simulink model "CanonicalMax"  (R2020a)
settings: Solver=VariableStepAuto  StartTime=0.0  StopTime=20  RelTol=1e-3
settings Model: Creator=Lenovo  LastModifiedBy=Lenovo

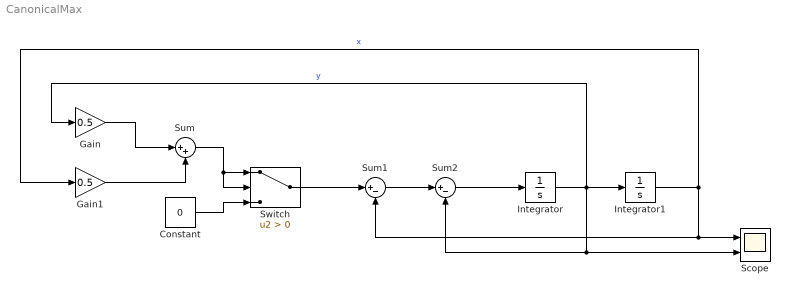
== system CanonicalMax ==
  Constant : Constant  Value=0
  Gain : Gain  Gain=0.5
  Gain1 : Gain  Gain=0.5
  Integrator : Integrator  InitialCondition=1
  Integrator1 : Integrator  InitialCondition=1
  Scope : Scope  NumInputPorts=2
  Sum : Sum  Inputs=|++
  Sum1 : Sum  Inputs=|+-
  Sum2 : Sum  Inputs=|+-
  Switch : Switch  Criteria=u2 > Threshold
  wires:
  Gain/1 -> Sum/1
  Gain1/1 -> Sum/2
  Sum1/1 -> Sum2/1
  Sum2/1 -> Integrator/1
  Integrator/1 -> Gain/1, Scope/2, Sum2/2, Integrator1/1  "y"
  Integrator1/1 -> Sum1/2, Scope/1, Gain1/1  "x"
  Sum/1 -> Switch/1, Switch/2
  Switch/1 -> Sum1/1
  Constant/1 -> Switch/3
